simulink model "DDC_Simulink_v2"  (R2025a)
settings: Solver=FixedStepDiscrete  StartTime=0.0  StopTime=5e-4  RelTol=1e-3
undefined symbols (not defined in the file): Add, h, Shift
libraries: dspsrcs4 x1, dsphdlsigops2 x1, dsphdlmathfun2 x1, dsphdlxfrm2 x1
settings Model: Creator=icemaster127  LastModifiedBy=icema

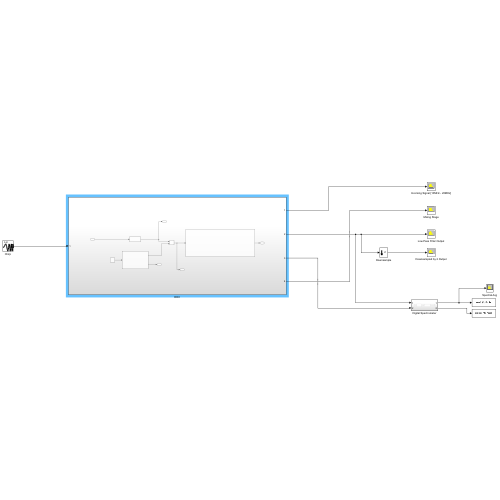
[thumbnail: Simulink's stored preview of the top-level diagram]
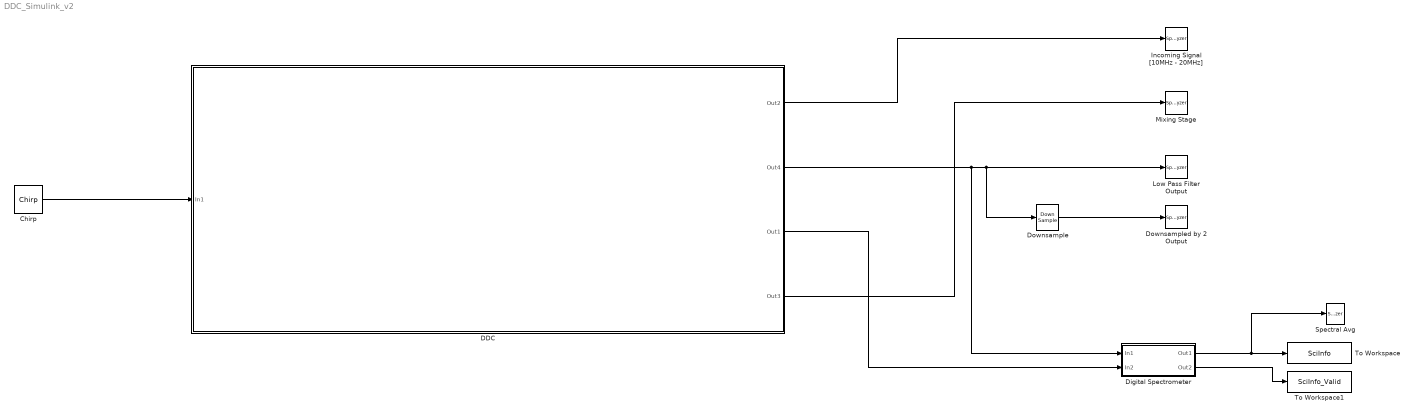
== system DDC_Simulink_v2 ==
  Chirp : dspsrcs4/Chirp  sweep=Linear  mode=Unidirectional  f0=10e6  f1=20e6  t1=.00001998  Tsweep=.00001998  phase=0  Ts=1/1/Fs  spf=1  datatype=double  OutputFrames=off
  DDC : Subsystem
  Digital Spectrometer : Subsystem
  Downsample : DownSample  RateOptions=Allow multirate processing
  Downsampled by 2 Output : SpectrumAnalyzer  WindowPosition=[433.000000,115.000000,354.000000,350.000000,]  Visible=on  ScopeFrameLocation=window  WindowInvariantSamplesPerUpdate=on  Span=30000000  StartFrequency=-15000000  StopFrequency=15000000  YLimits=[-42.8004 0.2334]
  Incoming Signal [10MHz - 20MHz] : SpectrumAnalyzer  WindowPosition=[7.000000,472.000000,425.000000,340.000000,]  Visible=on  ScopeFrameLocation=window  WindowInvariantSamplesPerUpdate=on  Span=60000000  StartFrequency=-30000000  StopFrequency=30000000  YLimits=[-36.4145 8.0975]  SelectedToolstripTab=spectrumAnalyzerToolstrip.spectralMaskTab
  Low Pass Filter Output : SpectrumAnalyzer  WindowPosition=[433.000000,495.000000,357.000000,317.000000,]  Visible=on  ScopeFrameLocation=window  WindowInvariantSamplesPerUpdate=on  YLimits=[-48.5586 2.8319]
  Mixing Stage : SpectrumAnalyzer  WindowPosition=[7.000000,119.000000,423.000000,322.000000,]  Visible=on  ScopeFrameLocation=window  WindowInvariantSamplesPerUpdate=on  YLimits=[-33.7411 0.7446]
  Spectral Avg : SpectrumAnalyzer  WindowPosition=[791.000000,508.000000,429.000000,304.000000,]  Visible=on  ScopeFrameLocation=window  WindowInvariantSamplesPerUpdate=on  YLimits=[-19.195 48.2732]
  To Workspace : ToWorkspace  VariableName=SciInfo  SampleTime=-1
      settings: Save2DSignal=2-D array (concatenate along first dimension)
  To Workspace1 : ToWorkspace  VariableName=SciInfo_Valid  SampleTime=-1
      settings: Save2DSignal=2-D array (concatenate along first dimension)
  wires:
  DDC/1(Out2) -> Incoming Signal [10MHz - 20MHz]/1
  DDC/4(Out3) -> Mixing Stage/1
  DDC/2(Out4) -> Digital Spectrometer/1(In1), Low Pass Filter Output/1, Downsample/1
  Chirp/1 -> DDC/1(In1)
  Downsample/1 -> Downsampled by 2 Output/1
  DDC/3(Out1) -> Digital Spectrometer/2(In2)
  Digital Spectrometer/1(Out1) -> Spectral Avg/1, To Workspace/1
  Digital Spectrometer/2(Out2) -> To Workspace1/1

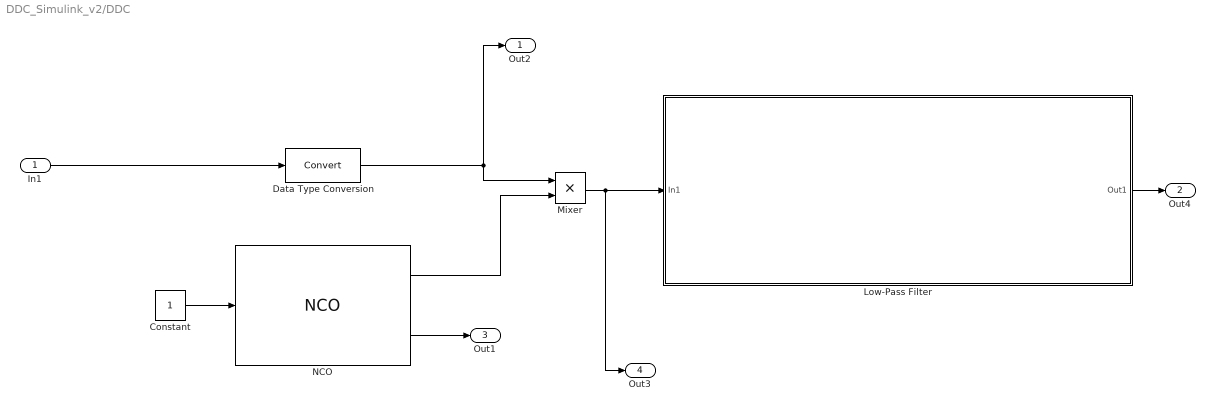
== system DDC_Simulink_v2/DDC ==
  In1 : Inport
  Constant : Constant  OutDataTypeStr=boolean
  Data Type Conversion : DataTypeConversion  SaturateOnIntegerOverflow=off  RndMeth=Floor
  Low-Pass Filter : Subsystem
  Mixer : Product
  NCO : dsphdlsigops2/NCO  PhaseIncrementSource=Property  PhaseIncrement=phIncr  PhaseOffsetSource=Property  PhaseOffset=phOff  DitherSource=Property  NumDitherBits=ditherBits  SamplesPerFrame=1  LUTCompress=off  ResetAction=off  Waveform=Cosine  PhasePort=off  SimulateUsing=Code generation  AccumulatorWL=32  PhaseQuantization=on  NumQuantizerAccumulatorBits=12  OutputDataType=Binary point scaling  OutputWL=16  OutputFL=14
      settings: LibrarySourceBlock=dsphdlsrcs2/NCO
  Out2 : Outport
  Out4 : Outport  Port=2
  Out1 : Outport  Port=3
  Out3 : Outport  Port=4
  wires:
  In1/1 -> Data Type Conversion/1
  Data Type Conversion/1 -> Out2/1, Mixer/1
  NCO/1 -> Mixer/2
  NCO/2 -> Out1/1
  Mixer/1 -> Out3/1, Low-Pass Filter/1(In1)
  Low-Pass Filter/1(Out1) -> Out4/1
  Constant/1 -> NCO/1

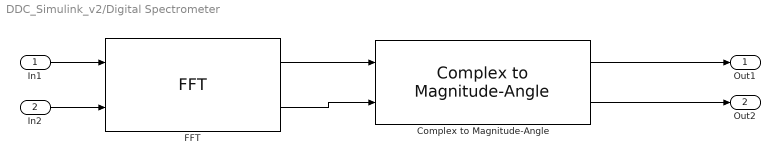
== system DDC_Simulink_v2/Digital Spectrometer ==
  In1 : Inport
  In2 : Inport  Port=2
  Complex to Magnitude-Angle : dsphdlmathfun2/Complex to Magnitude-Angle  NumIterationsSource=Auto  NumIterations=10  OutputFormat=Magnitude  AngleFormat=Normalized  ScaleOutput=on  ScalingMethod=Shift-Add  SimulateUsing=Code generation
  FFT : dsphdlxfrm2/FFT  Architecture=Streaming Radix 2^2  FFTLengthSource=Property  FFTLength=FFT  FFTLengthMax=1024  ComplexMultiplication=Use 4 multipliers and 2 adders  BitReversedOutput=off  BitReversedInput=off  Normalize=off  SimulateUsing=Code generation  RoundingMethod=Floor  ResetInputPort=off  StartOutputPort=off  EndOutputPort=off
  Out1 : Outport
  Out2 : Outport  Port=2
  wires:
  In2/1 -> FFT/2
  Complex to Magnitude-Angle/2 -> Out2/1
  FFT/1 -> Complex to Magnitude-Angle/1
  Complex to Magnitude-Angle/1 -> Out1/1
  In1/1 -> FFT/1
  FFT/2 -> Complex to Magnitude-Angle/2

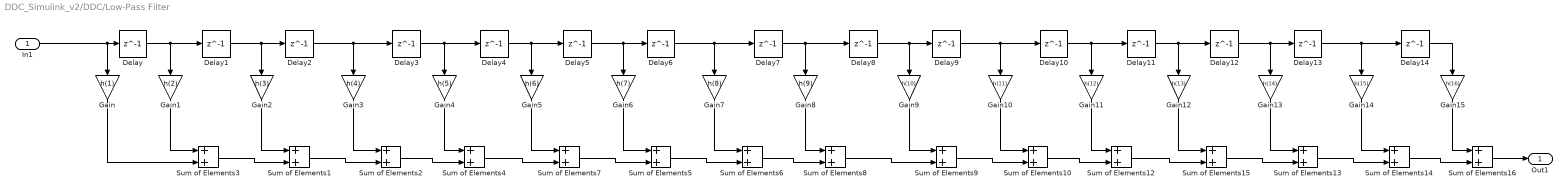
== system DDC_Simulink_v2/DDC/Low-Pass Filter ==
  In1 : Inport
  Delay{,1..14} (15 alike) : Delay  DelayLength=1
  Gain : Gain  Gain=h(1)
  Gain1 : Gain  Gain=h(2)
  Gain10 : Gain  Gain=h(11)
  Gain11 : Gain  Gain=h(12)
  Gain12 : Gain  Gain=h(13)
  Gain13 : Gain  Gain=h(14)
  Gain14 : Gain  Gain=h(15)
  Gain15 : Gain  Gain=h(16)
  Gain2 : Gain  Gain=h(3)
  Gain3 : Gain  Gain=h(4)
  Gain4 : Gain  Gain=h(5)
  Gain5 : Gain  Gain=h(6)
  Gain6 : Gain  Gain=h(7)
  Gain7 : Gain  Gain=h(8)
  Gain8 : Gain  Gain=h(9)
  Gain9 : Gain  Gain=h(10)
  Sum of Elements{1..10,12..16} (15 alike) : Sum
  Out1 : Outport
  wires:
  Delay1/1 -> Delay2/1, Gain2/1
  Delay/1 -> Delay1/1, Gain1/1
  In1/1 -> Gain/1, Delay/1
  Delay3/1 -> Delay4/1, Gain4/1
  Gain3/1 -> Sum of Elements2/1
  Delay2/1 -> Delay3/1, Gain3/1
  Sum of Elements1/1 -> Sum of Elements2/2
  Gain2/1 -> Sum of Elements1/1
  Sum of Elements3/1 -> Sum of Elements1/2
  Gain1/1 -> Sum of Elements3/1
  Gain/1 -> Sum of Elements3/2
  Gain4/1 -> Sum of Elements4/1
  Sum of Elements2/1 -> Sum of Elements4/2
  Sum of Elements5/1 -> Sum of Elements6/2
  Gain8/1 -> Sum of Elements8/1
  Delay6/1 -> Delay7/1, Gain7/1
  Delay4/1 -> Delay5/1, Gain5/1
  Delay5/1 -> Delay6/1, Gain6/1
  Delay7/1 -> Delay8/1, Gain8/1
  Sum of Elements7/1 -> Sum of Elements5/2
  Gain7/1 -> Sum of Elements6/1
  Gain5/1 -> Sum of Elements7/1
  Sum of Elements6/1 -> Sum of Elements8/2
  Gain6/1 -> Sum of Elements5/1
  Sum of Elements4/1 -> Sum of Elements7/2
  Gain14/1 -> Sum of Elements14/1
  Gain13/1 -> Sum of Elements13/1
  Sum of Elements9/1 -> Sum of Elements10/2
  Gain11/1 -> Sum of Elements12/1
  Gain12/1 -> Sum of Elements15/1
  Delay12/1 -> Delay13/1, Gain13/1
  Sum of Elements14/1 -> Sum of Elements16/2
  Delay11/1 -> Delay12/1, Gain12/1
  Gain15/1 -> Sum of Elements16/1
  Delay13/1 -> Delay14/1, Gain14/1
  Sum of Elements13/1 -> Sum of Elements14/2
  Delay9/1 -> Delay10/1, Gain10/1
  Delay8/1 -> Delay9/1, Gain9/1
  Gain10/1 -> Sum of Elements10/1
  Sum of Elements10/1 -> Sum of Elements12/2
  Sum of Elements12/1 -> Sum of Elements15/2
  Delay10/1 -> Delay11/1, Gain11/1
  Sum of Elements15/1 -> Sum of Elements13/2
  Gain9/1 -> Sum of Elements9/1
  Delay14/1 -> Gain15/1
  Sum of Elements8/1 -> Sum of Elements9/2
  Sum of Elements16/1 -> Out1/1
